simulink model "OMSdiag_bw"  (Simulink 7.0)
settings: Solver=ode4  SolverMode=SingleTasking  StartTime=0.0  StopTime=5  FixedStep=0.001  MaxStep=0.001  RelTol=1e-3  AbsTol=1e-3
undefined symbols (not defined in the file): cnsgain, LgtDrk, phasicgain, spgain, tonicgain
CloseFcn:
  | ;slview('closediagram',bdroot);
settings Model: Creator=jacobs  LastModifiedBy=lfd  ExtModeAutoUpdateStatusClock=off
settings DataIOCC: LimitDataPoints=off  SaveOutput=off  SaveTime=off
settings OptimizationCC: BlockReduction=off  BooleanDataType=off
settings DebuggingCC: SaveWithParameterizedLinksMsg=none  SignalResolutionControl=TryResolveAllWithWarning  SolverPrmCheckMsg=none  MultiTaskDSMMsg=warning  MultiTaskCondExecSysMsg=none  StrictBusMsg=None
settings HardwareCC: TargetUnknown=on
settings RTWCC: IncludeERTFirstTime=on
settings GRTTargetCC: TargetFcnLib=ansi_tfl_tmw.mat  ModelReferenceCompliant=off  MatFileLogging=off

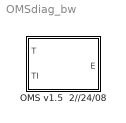
== system OMSdiag_bw ==
  OMS v1.5  2//24/08 : Subsystem
      mask init:
      | k=0.25;loadmdlp;prolong_buffersize=5120;
      mask Display: disp('OMS v1.5\nModel')

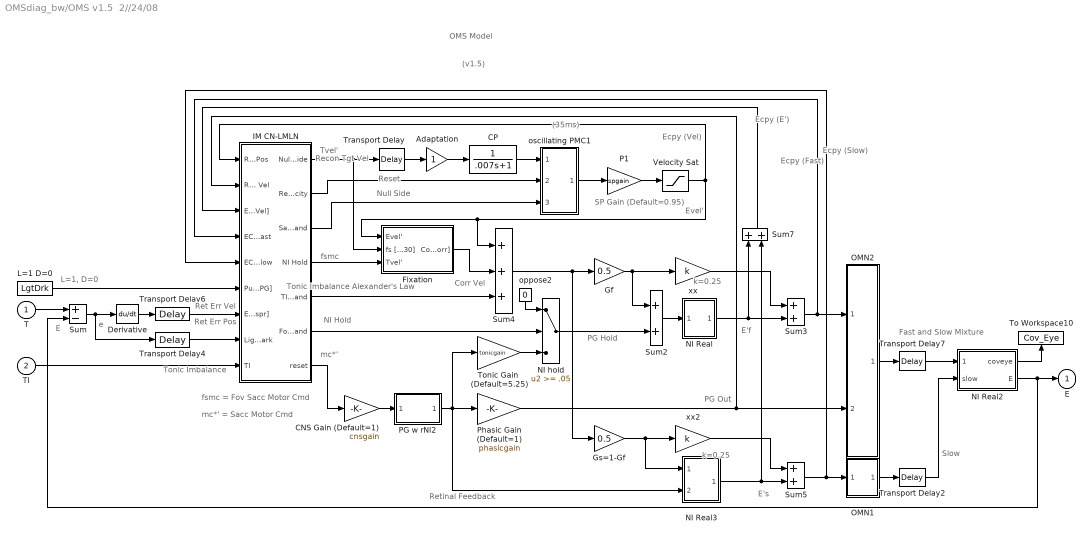
== system OMSdiag_bw/OMS v1.5  2//24/08 ==
  note: E'f
  note: k=0.25
  note: E
  note: e
  note: Tonic Imbalance
      | Alexander's Law
  note: NI Hold
  note: mc*'
  note: Tvel'
  note: Ecpy
      | (E')
  note: Ecpy (Vel)
  note: (35ms)
  note: Retinal Feedback
  note: Recon Tgt Vel
  note: Evel'
  note: OMS Model
  note: Ecpy
      | (Fast)
  note: Ret Err Vel
  note: SP Gain
      | (Default=0.95)
  note: L=1, D=0
  note: Corr Vel
  note: fsmc
  note: Null Side
  note: k=0.25
  note: Fast and Slow
      | Mixture
  note: Slow
  note: Ecpy
      | (Slow)
  note: Reset
  note: E's
  note: PG Out
  note: Ret Err Pos
  note: Tonic Imbalance
  note: fsmc = Fov Sacc Motor Cmd
  note: mc*' = Sacc Motor Cmd
  note: (v1.5)
  note: PG Hold
  T : Inport  OutDataType=sfix(16)  OutScaling=2^0
  TI : Inport  Port=2  OutDataType=sfix(16)  OutScaling=2^0
  Adaptation : Gain  ParameterDataType=sfix(16)  ParameterScaling=2^0  OutDataType=sfix(16)  OutScaling=2^0  SaturateOnIntegerOverflow=on
  CNS Gain (Default=1) : Gain  Gain=cnsgain  ParameterDataType=sfix(16)  ParameterScaling=2^0  OutDataType=sfix(16)  OutScaling=2^0  SaturateOnIntegerOverflow=on
  CP : TransferFcn  Denominator=[.007 1]
  Derivative : Derivative
      mask Display: disp('s')
  Fixation : Subsystem
      mask Display: disp('Fixation')
  Gf : Gain  Gain=0.5  ParameterDataType=sfix(16)  ParameterScaling=2^0  OutDataType=sfix(16)  OutScaling=2^0  SaturateOnIntegerOverflow=on
  Gs=1-Gf : Gain  Gain=0.5  ParameterDataType=sfix(16)  ParameterScaling=2^0  OutDataType=sfix(16)  OutScaling=2^0  SaturateOnIntegerOverflow=on
  IM CN-LMLN : Subsystem
      mask Display: disp('INTERNAL\nMONITOR')
  L=1 D=0 : Constant  Value=LgtDrk  OutDataType=sfix(16)  OutScaling=2^0
  NI Real : Subsystem
      mask Display: disp('NI\n(Fast)')
  NI Real2 : Subsystem
      mask Display: disp('Plant')
  NI Real3 : Subsystem
      mask Display: disp('rNI\n(Slow)')
  NI hold : Switch  Threshold=.05  SaturateOnIntegerOverflow=on  InputSameDT=on
  OMN1 : Subsystem
      mask Display: disp('OMN\n(Slow)')
  OMN2 : Subsystem
      mask Display: disp('OMN\n(Fast)')
  P1 : Gain  Gain=spgain  ParameterDataType=sfix(16)  ParameterScaling=2^0  OutDataType=sfix(16)  OutScaling=2^0  SaturateOnIntegerOverflow=on
  PG w rNI2 : Subsystem
      mask Display: disp('PG rNI 2\n(2P)')
  Phasic Gain (Default=1) : Gain  Gain=phasicgain  ParameterDataType=sfix(16)  ParameterScaling=2^0  OutDataType=sfix(16)  OutScaling=2^0  SaturateOnIntegerOverflow=on
  Sum : Sum  Inputs=+-  OutDataType=sfix(16)  OutScaling=2^0  SaturateOnIntegerOverflow=on  InputSameDT=on
  Sum2 : Sum  OutDataType=sfix(16)  OutScaling=2^0  SaturateOnIntegerOverflow=on  InputSameDT=on
  Sum3 : Sum  OutDataType=sfix(16)  OutScaling=2^0  SaturateOnIntegerOverflow=on  InputSameDT=on
  Sum4 : Sum  Inputs=+++  OutDataType=sfix(16)  OutScaling=2^0  SaturateOnIntegerOverflow=on  InputSameDT=on
  Sum5 : Sum  OutDataType=sfix(16)  OutScaling=2^0  SaturateOnIntegerOverflow=on  InputSameDT=on
  Sum7 : Sum  Orientation=up  OutDataType=sfix(16)  OutScaling=2^0  SaturateOnIntegerOverflow=on  InputSameDT=on
  To Workspace10 : ToWorkspace  VariableName=Cov_Eye  SaveFormat=Array
      settings: Orientation=up  MaxDataPoints=10000
  Tonic Gain  (Default=5.25) : Gain  Gain=tonicgain  ParameterDataType=sfix(16)  ParameterScaling=2^0  OutDataType=sfix(16)  OutScaling=2^0  SaturateOnIntegerOverflow=on
  Transport Delay : TransportDelay  DelayTime=0.015
      mask Display: disp('15ms')
  Transport Delay2 : TransportDelay  DelayTime=0.005
      mask Display: disp('5ms')
  Transport Delay4 : TransportDelay  DelayTime=.05
      mask Display: disp('50ms')
  Transport Delay6 : TransportDelay  DelayTime=.05
      mask Display: disp('50ms')
  Transport Delay7 : TransportDelay  DelayTime=0.005
      mask Display: disp('5ms')
  Velocity Sat : Saturate  UpperLimit=90  LowerLimit=-90
  oppose2 : Constant  Orientation=down  Value=0  OutDataType=sfix(16)  OutScaling=2^0
  oscillating PMC1 : Subsystem
      mask Display: disp('PMC+')
  xx : Gain  Gain=k  ParameterDataType=sfix(16)  ParameterScaling=2^0  OutDataType=sfix(16)  OutScaling=2^0  SaturateOnIntegerOverflow=on
  xx2 : Gain  Gain=k  ParameterDataType=sfix(16)  ParameterScaling=2^0  OutDataType=sfix(16)  OutScaling=2^0  SaturateOnIntegerOverflow=on
  E : Outport  OutDataType=sfix(16)  OutScaling=2^0  InitialOutput=0
  wires:
  Derivative/1 -> Transport Delay6/1
  Sum/1 -> Derivative/1, Transport Delay4/1
  CP/1 -> oscillating PMC1/1(desired eye vel)
  oscillating PMC1/1(efference copy eye vel) -> P1/1
  Transport Delay/1 -> Adaptation/1
  Velocity Sat/1 -> Fixation/1(Evel'), Sum4/1, IM CN-LMLN/1(RetErr Pos)
  P1/1 -> Velocity Sat/1
  PG w rNI2/1(PG [pgout]) -> Tonic Gain  (Default=5.25)/1, Phasic Gain (Default=1)/1, NI Real3/2(PG + (TIAL+SP)1)
  Tonic Gain  (Default=5.25)/1 -> NI hold/3
  xx/1 -> Sum3/1
  NI Real/1(NIOUT [epospr]) -> Sum3/2, Sum7/1
  Sum3/1 -> OMN2/1("[eposspf]"), IM CN-LMLN/4(ECPY Fast)
  oppose2/1 -> NI hold/1
  CNS Gain (Default=1)/1 -> PG w rNI2/1("[mcsprd]")
  Sum2/1 -> NI Real/1(PG + (TIAL+SP))
  OMN2/1("[psout]") -> Transport Delay7/1
  xx2/1 -> Sum5/1
  NI Real3/1(NIOUT [epospr]) -> Sum5/2, Sum7/2
  Transport Delay2/1 -> NI Real2/2(slow)
  Sum5/1 -> OMN1/1("[epossps] "), IM CN-LMLN/5(ECPY Slow)
  OMN1/1("  [sout] ") -> Transport Delay2/1
  Transport Delay7/1 -> NI Real2/1("   ")
  NI Real2/1(coveye) -> To Workspace10/1
  NI Real2/2(E) -> E/1, Sum/2
  Gf/1 -> xx/1, Sum2/1
  NI hold/1 -> Sum2/2
  Adaptation/1 -> CP/1
  Phasic Gain (Default=1)/1 -> IM CN-LMLN/2(RetErr Vel), OMN2/2("[pgout]")
  TI/1 -> IM CN-LMLN/9(TI)
  Transport Delay4/1 -> IM CN-LMLN/8(Light /Dark)
  Transport Delay6/1 -> IM CN-LMLN/7(ECPY [epospr])
  T/1 -> Sum/1
  IM CN-LMLN/7(reset) -> CNS Gain (Default=1)/1
  IM CN-LMLN/6(Foveating Saccade Motor Command) -> NI hold/2
  IM CN-LMLN/1(Null Side) -> Transport Delay/1, Fixation/2(fs [fsmc30])
  IM CN-LMLN/2(Reconstructed Target Velocity) -> oscillating PMC1/2(fpmc)
  IM CN-LMLN/3(Saccadic Motor Command) -> oscillating PMC1/3(null side)
  IM CN-LMLN/4(NI Hold) -> Fixation/3(Tvel')
  IM CN-LMLN/5(TIAL Motor Command) -> Sum4/3
  Fixation/1(" CorrVel [velcorr]") -> Sum4/2
  Sum4/1 -> Gf/1, Gs=1-Gf/1
  Sum7/1 -> IM CN-LMLN/3(ECPY [Vel])
  L=1 D=0/1 -> IM CN-LMLN/6(Pulse Gen [PG])
  Gs=1-Gf/1 -> xx2/1, NI Real3/1(PG + (TIAL+SP))

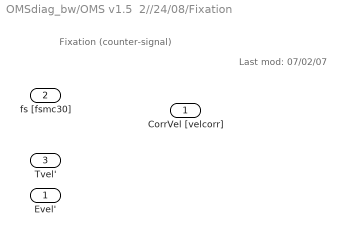
== system OMSdiag_bw/OMS v1.5  2//24/08/Fixation ==
  note: Fixation (counter-signal)
  note: Last mod: 07/02/07
  Evel' : Inport  OutDataType=sfix(16)  OutScaling=2^0
  fs [fsmc30] : Inport  Port=2  OutDataType=sfix(16)  OutScaling=2^0
  Tvel' : Inport  Port=3  OutDataType=sfix(16)  OutScaling=2^0
  " CorrVel [velcorr]" : Outport  OutDataType=sfix(16)  OutScaling=2^0  InitialOutput=0

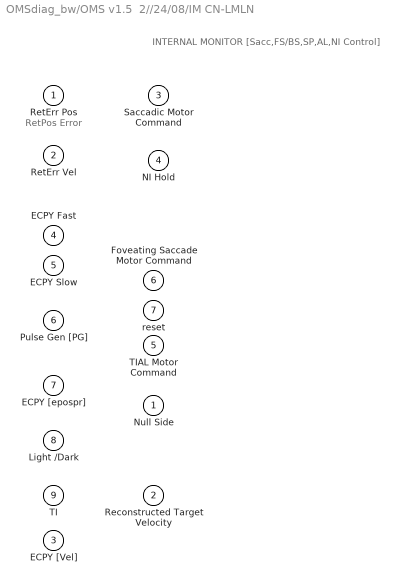
== system OMSdiag_bw/OMS v1.5  2//24/08/IM CN-LMLN ==
  note: INTERNAL MONITOR [Sacc,FS/BS,SP,AL,NI Control]
  note: RetPos
      | Error
  RetErr Pos : Inport  OutDataType=sfix(16)  OutScaling=2^0
  RetErr Vel : Inport  Port=2  OutDataType=sfix(16)  OutScaling=2^0
  ECPY [Vel] : Inport  Port=3  OutDataType=sfix(16)  OutScaling=2^0
  ECPY Fast : Inport  Port=4  OutDataType=sfix(16)  OutScaling=2^0
  ECPY Slow : Inport  Port=5  OutDataType=sfix(16)  OutScaling=2^0
  Pulse Gen [PG] : Inport  Port=6  OutDataType=sfix(16)  OutScaling=2^0
  ECPY [epospr] : Inport  Port=7  OutDataType=sfix(16)  OutScaling=2^0
  Light /Dark : Inport  Port=8  OutDataType=sfix(16)  OutScaling=2^0
  TI : Inport  Port=9  OutDataType=sfix(16)  OutScaling=2^0
  Null Side : Outport  OutDataType=sfix(16)  OutScaling=2^0  InitialOutput=0
  Reconstructed Target Velocity : Outport  Port=2  OutDataType=sfix(16)  OutScaling=2^0  InitialOutput=0
  Saccadic Motor Command : Outport  Port=3  OutDataType=sfix(16)  OutScaling=2^0  InitialOutput=0
  NI Hold : Outport  Port=4  OutDataType=sfix(16)  OutScaling=2^0  InitialOutput=0
  TIAL Motor Command : Outport  Port=5  OutDataType=sfix(16)  OutScaling=2^0  InitialOutput=0
  Foveating Saccade Motor Command : Outport  Port=6  OutDataType=sfix(16)  OutScaling=2^0  InitialOutput=0
  reset : Outport  Port=7  OutDataType=sfix(16)  OutScaling=2^0  InitialOutput=0

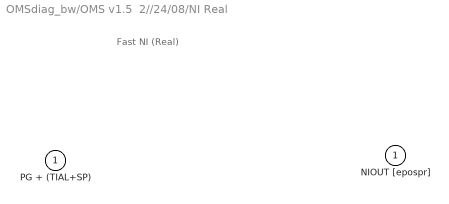
== system OMSdiag_bw/OMS v1.5  2//24/08/NI Real ==
  note: Fast NI (Real)
  PG + (TIAL+SP) : Inport  OutDataType=sfix(16)  OutScaling=2^0
  NIOUT [epospr] : Outport  OutDataType=sfix(16)  OutScaling=2^0  InitialOutput=0

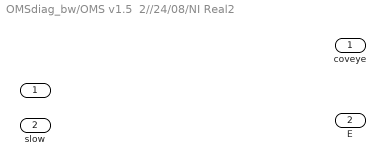
== system OMSdiag_bw/OMS v1.5  2//24/08/NI Real2 ==
  "   " : Inport  OutDataType=sfix(16)  OutScaling=2^0
  slow : Inport  Port=2  OutDataType=sfix(16)  OutScaling=2^0
  coveye : Outport  OutDataType=sfix(16)  OutScaling=2^0
  E : Outport  Port=2  OutDataType=sfix(16)  OutScaling=2^0
  wires:
  ? -> coveye/1
  ? -> E/1

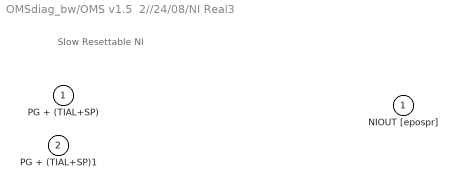
== system OMSdiag_bw/OMS v1.5  2//24/08/NI Real3 ==
  note: Slow Resettable NI
  PG + (TIAL+SP) : Inport  OutDataType=sfix(16)  OutScaling=2^0
  PG + (TIAL+SP)1 : Inport  Port=2  OutDataType=sfix(16)  OutScaling=2^0
  NIOUT [epospr] : Outport  OutDataType=sfix(16)  OutScaling=2^0  InitialOutput=0

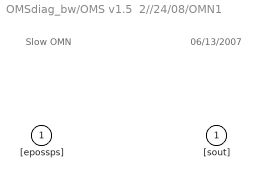
== system OMSdiag_bw/OMS v1.5  2//24/08/OMN1 ==
  note: Slow OMN
  note: 06/13/2007
  "[epossps] " : Inport  OutDataType=sfix(16)  OutScaling=2^0
  "  [sout] " : Outport  OutDataType=sfix(16)  OutScaling=2^0  InitialOutput=0

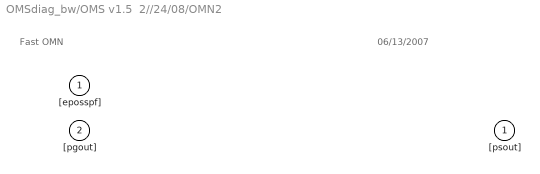
== system OMSdiag_bw/OMS v1.5  2//24/08/OMN2 ==
  note: Fast OMN
  note: 06/13/2007
  "[eposspf]" : Inport  OutDataType=sfix(16)  OutScaling=2^0
  "[pgout]" : Inport  Port=2  OutDataType=sfix(16)  OutScaling=2^0
  "[psout]" : Outport  OutDataType=sfix(16)  OutScaling=2^0  InitialOutput=0

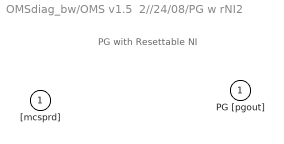
== system OMSdiag_bw/OMS v1.5  2//24/08/PG w rNI2 ==
  note: PG with Resettable NI
  "[mcsprd]" : Inport  OutDataType=sfix(16)  OutScaling=2^0
  PG [pgout] : Outport  OutDataType=sfix(16)  OutScaling=2^0  InitialOutput=0

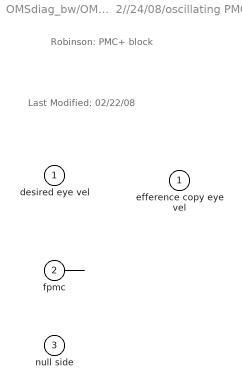
== system OMSdiag_bw/OMS v1.5  2//24/08/oscillating PMC1 ==
  note: Last Modified:
      | 02/22/08
  note: Robinson: PMC+ block
  desired eye vel : Inport  OutDataType=sfix(16)  OutScaling=2^0
  fpmc : Inport  Port=2  OutDataType=sfix(16)  OutScaling=2^0
  null side : Inport  Port=3  OutDataType=sfix(16)  OutScaling=2^0
  efference copy eye vel : Outport  OutDataType=sfix(16)  OutScaling=2^0  InitialOutput=0
  wires:
  fpmc/1 -> ?
